simulink model "optimis_crane_2_vanilla"  (R2016b)
settings: Solver=FixedStepAuto  StartTime=0.0  StopTime=inf  FixedStep=0.01  RelTol=1e-3
undefined symbols (not defined in the file): Kd, Kdx, Ki, Kix, Kp, Kpx, M, m, MR, Nx, Ny, start_course, TorqueMultX, TorqueMultY, TorqueMultZ, total_waypoints, TxBreak, TxCoulomb, TxTrans, TxVisc, TyBreak, TyCoulomb, TyTrans, TyVisc, TzBreak, TzCoulomb, TzTrans, TzVisc, X, xRange, xwaypoints, xZero, Y, yRange, ywaypoints, yZero, Z, zRange, zZero
libraries: sm_lib x146, fl_lib x62, nesl_utility x24, elec_lib x9, simulink x8, sm_double_wishbone_suspension_lib x4, checkpacklib x2, aerolibtransform2 x1
(part 1 of 14)
settings Model: Creator=nadeen  LastModifiedBy=nadeen
settings DataIOCC: ReturnWorkspaceOutputs=on

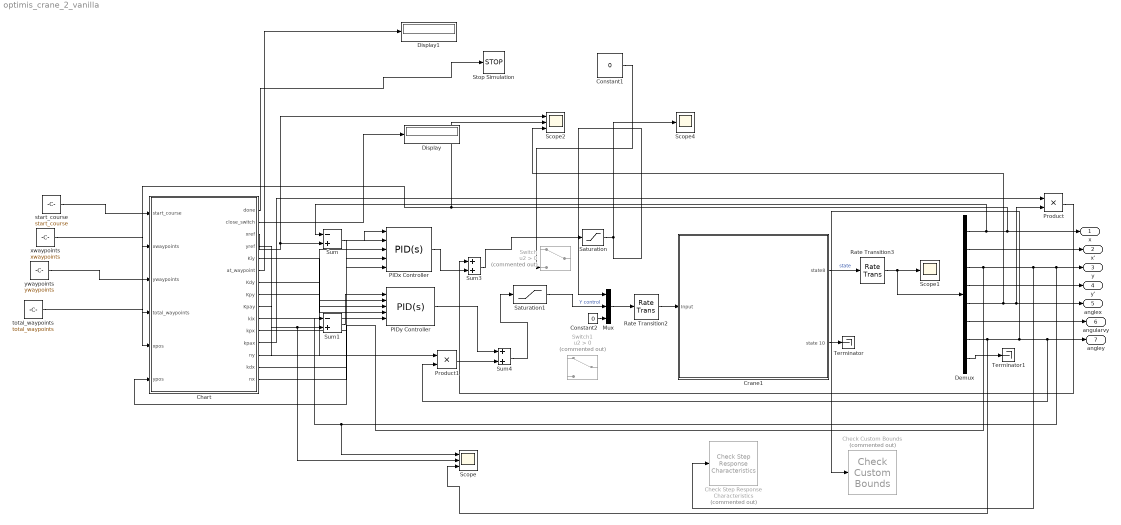
== system optimis_crane_2_vanilla ==
  Chart : Stateflow chart  TreatAsAtomicUnit=on
  Check Custom Bounds : checkpacklib/Check Custom Bounds  Commented=on  InstantiateOnLoad=on  enabled=on  stopWhenAssertionFail=off  export=off  ViewDlgPos=[]  OpenViewOnLoad=off  LaunchViewOnOpen=off  TimeUnits=seconds  EnableUpperBound=on  UpperBoundTimes="[0  2.5;2.5 5.99]"  UpperBoundAmplitudes=[0.15 0.15; 0.02 0.020];  EnableLowerBound=on  LowerBoundTimes="[0  2.5 ; 2.5 5.99]"  LowerBoundAmplitudes=[-0.15 -0.15; -0.02 -0.02];
  Check Step Response Characteristics : checkpacklib/Check Step Response  Characteristics  Commented=on  InstantiateOnLoad=on  enabled=on  stopWhenAssertionFail=off  export=off  ViewDlgPos=[]  OpenViewOnLoad=off  LaunchViewOnOpen=off  TimeUnits=seconds  EnableStepResponseBound=on  InitialValue=0  FinalValue=0.01  StepTime=0  RiseTime=2.5  PercentRise=60  SettlingTime=3  PercentSettling=40  PercentOvershoot=90  PercentUndershoot=90
  Constant1 : Constant  Value=0  VectorParams1D=off  SampleTime=-1
  Constant2 : Constant  Value=0
  Crane1 : Subsystem  mask{penduMass=m, cartMass=M, MR=MR, xRange=xRange, yRange=yRange, zRange=zRange, xZero=xZero, yZero=yZero, zZero=zZero, TxBreak=TxBreak, TxCoulomb=TxCoulomb, TxVisc=TxVisc, TxTrans=TxTrans, TyBreak=TyBreak, TyCoulomb=TyCoulomb, TyVisc=TyVisc, TyTrans=TyTrans, TzBreak=TzBreak, TzCoulomb=TzCoulomb, TzVisc=TzVisc, TzTrans=TzTrans, Ux=TorqueMultX, Uy=TorqueMultY, Uz=TorqueMultZ}
      mask prompts: penduMass "Pendulum Mass (Kg)"; cartMass "Mass of the cart (Kg)"; MR "Mass of the rail (Kg)"; TxBreak "BreakAwayFriction"; TxCoulomb "Coulomb Friction"; TxVisc "Viscous friction"; TxTrans "Transition coeff"; TyBreak "BreakAwayFriction"; TyCoulomb "Coulomb Friction"; TyVisc "Viscous friction"; TyTrans "Transition coeff"; TzBreak "BreakAwayFriction"; TzCoulomb "Coulomb Friction"; TzVisc "Viscous friction"; TzTrans "Transition coeff"; Ux "Rail motor multiplier (X)"; Uy "Cart motor multiplier (Y)"; Uz "String motor multiplier (Z)"
      mask init:
      | %mass lowSat
      | penduMass=max(penduMass,1e-3);
      | cartMass=max(cartMass,1e-3);
      | MR=max(MR,1e-3);
      | 
      | %zeros saturated
      | xZero=max(xZero,xRange(1));
      | xZero=min(xZero,xRange(2));
      | 
      | yZero=max(yZero,yRange(1));
      | yZero=min(yZero,yRange(2));
      | 
      | zZero=max(zZero,zRange(1));
      | zZero=min(zZero,zRange(2));
      mask DialogControl DescGroupVar Prompt: 3D Crane Simscape model
      mask Display:
